simulink model "Simulink_Linear_Module_2"  (R2019b)
settings: Solver=VariableStepAuto  StartTime=0.0  StopTime=6  RelTol=1e-3
settings Model: Creator=rjgoo  LastModifiedBy=rjgoo
settings DataIOCC: ReturnWorkspaceOutputs=off
settings DebuggingCC: ArithmeticOperatorsInVariantConditions=warning
settings SFSimCC: SimUseLocalCustomCode=off  CustomCodeUndefinedFunction=UseInterfaceOnly
settings RTWCC: RTWUseLocalCustomCode=off

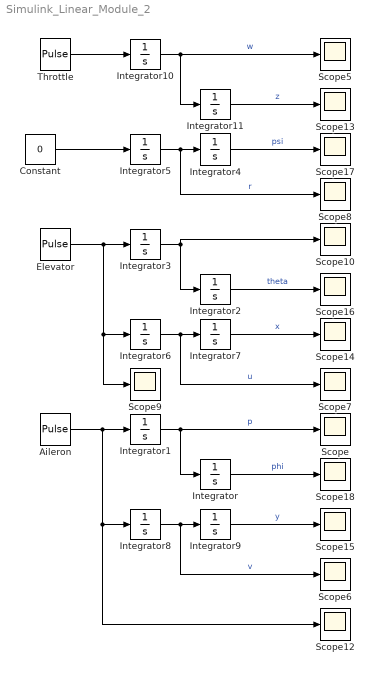
== system Simulink_Linear_Module_2 ==
  " Throttle" : DiscretePulseGenerator  PulseType=Time based  Amplitude=0  Period=8  PulseWidth=50  PhaseDelay=1
  Aileron : DiscretePulseGenerator  PulseType=Time based  Amplitude=0.1  Period=8  PulseWidth=50  PhaseDelay=1
  Constant : Constant  Value=0
  Elevator : DiscretePulseGenerator  PulseType=Time based  Amplitude=0  Period=80  PulseWidth=50  PhaseDelay=1
  Integrator{,1..11} (12 alike) : Integrator
  Scope{,5..10,12..18} (14 alike) : Scope
  wires:
  Aileron/1 -> Scope12/1, Integrator8/1, Integrator1/1
  Integrator11/1 -> Scope13/1  "z"
  Integrator5/1 -> Integrator4/1, Scope8/1  "r"
  Integrator/1 -> Scope18/1  "phi"
  Integrator4/1 -> Scope17/1  "psi"
  Integrator9/1 -> Scope15/1  "y"
  " Throttle"/1 -> Integrator10/1
  Integrator3/1 -> Integrator2/1, Scope10/1
  Integrator2/1 -> Scope16/1  "theta"
  Integrator7/1 -> Scope14/1  "x"
  Integrator1/1 -> Integrator/1, Scope/1  "p"
  Constant/1 -> Integrator5/1
  Integrator6/1 -> Integrator7/1, Scope7/1  "u"
  Integrator8/1 -> Scope6/1, Integrator9/1  "v"
  Integrator10/1 -> Integrator11/1, Scope5/1  "w"
  Elevator/1 -> Scope9/1, Integrator6/1, Integrator3/1
